simulink model "closedloop_saturation1"  (R2018a)
settings: Solver=ode23t  StartTime=0.0  StopTime=5  MaxStep=0.01  RelTol=1e-3
InitFcn:
  | % stop_time_as_str = get_param(gcs, 'StopTime');
  | % T= str2double(stop_time_as_str);
model workspace (MATLAB code in the model file):
  | % Simscape(TM) Multibody(TM) version: 7.1
  | 
  | % This is a model data file derived from a Simscape Multibody Import XML file using the smimport function.
  | % The data in this file sets the block parameter values in an imported Simscape Multibody model.
  | % For more information on this file, see the smimport function help page in the Simscape Multibody documentation.
  | % You can modify numerical values, but avoid any other changes to this file.
  | % Do not add code to this file. Do not edit the physical units shown in comments.
  | 
  | %%%VariableName:smiData
  | 
  | 
  | %============= RigidTransform =============%
  | 
  | %Initialize the RigidTransform structure array by filling in null values.
  | smiData.RigidTransform(23).translation = [0.0 0.0 0.0];
  | smiData.RigidTransform(23).angle = 0.0;
  | smiData.RigidTransform(23).axis = [0.0 0.0 0.0];
  | smiData.RigidTransform(23).ID = '';
  | 
  | %Translation Method - Cartesian
  | %Rotation Method - Arbitrary Axis
  | smiData.RigidTransform(1).translation = [0 0 20];  % mm
  | smiData.RigidTransform(1).angle = 3.1415926535897931;  % rad
  | smiData.RigidTransform(1).axis = [1 0 0];
  | smiData.RigidTransform(1).ID = 'B[Base-1:-:Plane-1]';
  | 
  | %Translation Method - Cartesian
  | %Rotation Method - Arbitrary Axis
  | smiData.RigidTransform(2).translation = [0 -280 30];  % mm
  | smiData.RigidTransform(2).angle = 3.1415926535897931;  % rad
  | smiData.RigidTransform(2).axis = [1 0 0];
  | smiData.RigidTransform(2).ID = 'F[Base-1:-:Plane-1]';
  | 
  | %Translation Method - Cartesian
  | %Rotation Method - Arbitrary Axis
  | smiData.RigidTransform(3).translation = [-650 -399.99999999999994 10];  % mm
  | smiData.RigidTransform(3).angle = 2.0943951023931953;  % rad
  | smiData.RigidTransform(3).axis = [0.57735026918962584 -0.57735026918962584 0.57735026918962584];
  | smiData.RigidTransform(3).ID = 'B[Plane-1:-:]';
  | 
  | %Translation Method - Cartesian
  | %Rotation Method - Arbitrary Axis
  | smiData.RigidTransform(4).translation = [-650 -119.99999999999994 0];  % mm
  | smiData.RigidTransform(4).angle = 2.0943951023931953;  % rad
  | smiData.RigidTransform(4).axis = [0.57735026918962584 -0.57735026918962584 0.57735026918962584];
  | smiData.RigidTransform(4).ID = 'F[Plane-1:-:]';
  | 
  | %Translation Method - Cartesian
  | %Rotation Method - Arbitrary Axis
  | smiData.RigidTransform(5).translation = [0 -20 60];  % mm
  | smiData.RigidTransform(5).angle = 2.0943951023931953;  % rad
  | smiData.RigidTransform(5).axis = [-0.57735026918962584 -0.57735026918962584 -0.57735026918962584];
  | smiData.RigidTransform(5).ID = 'B[Link1-1:-:Link2-1]';
  | 
  | %Translation Method - Cartesian
  | %Rotation Method - Arbitrary Axis
  | smiData.RigidTransform(6).translation = [20.000000000000004 -6.8922645368729718e-13 -40.000000000002252];  % mm
  | smiData.RigidTransform(6).angle = 2.0943951023931957;  % rad
  | smiData.RigidTransform(6).axis = [-0.57735026918962573 -0.57735026918962562 0.57735026918962573];
  | smiData.RigidTransform(6).ID = 'F[Link1-1:-:Link2-1]';
  | 
  | %Translation Method - Cartesian
  | %Rotation Method - Arbitrary Axis
  | smiData.RigidTransform(7).translation = [0 0 110.00000000000001];  % mm
  | smiData.RigidTransform(7).angle = 0;  % rad
  | smiData.RigidTransform(7).axis = [0 0 0];
  | smiData.RigidTransform(7).ID = 'B[Base-1:-:Link1-1]';
  | 
  | %Translation Method - Cartesian
  | %Rotation Method - Arbitrary Axis
  | smiData.RigidTransform(8).translation = [0 0 -2.8421709430404007e-14];  % mm
  | smiData.RigidTransform(8).angle = 0;  % rad
  | smiData.RigidTransform(8).axis = [0 0 0];
  | smiData.RigidTransform(8).ID = 'F[Base-1:-:Link1-1]';
  | 
  | %Translation Method - Cartesian
  | %Rotation Method - Arbitrary Axis
  | smiData.RigidTransform(9).translation = [-7 0 260];  % mm
  | smiData.RigidTransform(9).angle = 2.0943951023931953;  % rad
  | smiData.RigidTransform(9).axis = [0.57735026918962584 0.57735026918962584 0.57735026918962584];
  | smiData.RigidTransform(9).ID = 'B[Link2-1:-:Link3-1]';
  | 
  | %Translation Method - Cartesian
  | %Rotation Method - Arbitrary Axis
  | smiData.RigidTransform(10).translation = [7.0000000000000213 2.4034108037085389e-12 -40.000000000000242];  % mm
  | smiData.RigidTransform(10).angle = 2.0943951023931957;  % rad
  | smiData.RigidTransform(10).axis = [-0.57735026918962595 -0.57735026918962573 0.57735026918962551];
  | smiData.RigidTransform(10).ID = 'F[Link2-1:-:Link3-1]';
  | 
  | %Translation Method - Cartesian
  | %Rotation Method - Arbitrary Axis
  | smiData.RigidTransform(11).translation = [-12 0 220];  % mm
  | smiData.RigidTransform(11).angle = 2.0943951023931953;  % rad
  | smiData.RigidTransform(11).axis = [0.57735026918962584 0.57735026918962584 0.57735026918962584];
  | smiData.RigidTransform(11).ID = 'B[Link3-1:-:Link4-1]';
  | 
  | %Translation Method - Cartesian
  | %Rotation Method - Arbitrary Axis
  | smiData.RigidTransform(12).translation = [11.999999999999968 -3.5527136788005009e-14 -29.999999999999815];  % mm
  | smiData.RigidTransform(12).angle = 2.0943951023931957;  % rad
  | smiData.RigidTransform(12).axis = [-0.57735026918962573 -0.57735026918962573 0.57735026918962562];
  | smiData.RigidTransform(12).ID = 'F[Link3-1:-:Link4-1]';
  | 
  | %Translation Method - Cartesian
  | %Rotation Method - Arbitrary Axis
  | smiData.RigidTransform(13).translation = [0 0 0];  % mm
  | smiData.RigidTransform(13).angle = 0;  % rad
  | smiData.RigidTransform(13).axis = [0 0 0];
  | smiData.RigidTransform(13).ID = 'B[Base-1:-:]';
  | 
  | %Translation Method - Cartesian
  | %Rotation Method - Arbitrary Axis
  | smiData.RigidTransform(14).translation = [0 0 0];  % mm
  | smiData.RigidTransform(14).angle = 0;  % rad
  | smiData.RigidTransform(14).axis = [0 0 0];
  | smiData.RigidTransform(14).ID = 'F[Base-1:-:]';
  | 
  | %Translation Method - Cartesian
  | %Rotation Method - Arbitrary Axis
  | smiData.RigidTransform(15).translation = [0 1.1102230246251565e-13 20.000000000000018];  % mm
  | smiData.RigidTransform(15).angle = 0;  % rad
  | smiData.RigidTransform(15).axis = [0 0 0];
  | smiData.RigidTransform(15).ID = 'B[Link4-1:-:Tool1-1]';
  | 
  | %Translation Method - Cartesian
  | %Rotation Method - Arbitrary Axis
  | smiData.RigidTransform(16).translation = [2.4922286456785514e-12 -4.9999999999999751 1.2168044349891716e-13];  % mm
  | smiData.RigidTransform(16).angle = 2.0943951023931957;  % rad
  | smiData.RigidTransform(16).axis = [-0.57735026918962595 -0.57735026918962573 -0.57735026918962551];
  | smiData.RigidTransform(16).ID = 'F[Link4-1:-:Tool1-1]';
  | 
  | %Translation Method - Cartesian
  | %Rotation Method - Arbitrary Axis
  | smiData.RigidTransform(17).translation = [-40.385164807134494 17.000000000000028 2.5000000000000022];  % mm
  | smiData.RigidTransform(17).angle = 2.0943951023931953;  % rad
  | smiData.RigidTransform(17).axis = [0.57735026918962584 0.57735026918962584 0.57735026918962584];
  | smiData.RigidTransform(17).ID = 'B[Tool1-1:-:Tool2-1]';
  | 
  | %Translation Method - Cartesian
  | %Rotation Method - Arbitrary Axis
  | smiData.RigidTransform(18).translation = [-2.4999999999999627 10.385164807134508 -17.999999999999989];  % mm
  | smiData.RigidTransform(18).angle = 2.0943951023931957;  % rad
  | smiData.RigidTransform(18).axis = [0.57735026918962573 -0.57735026918962573 0.57735026918962562];
  | smiData.RigidTransform(18).ID = 'F[Tool1-1:-:Tool2-1]';
  | 
  | %Translation Method - Cartesian
  | %Rotation Method - Arbitrary Axis
  | smiData.RigidTransform(19).translation = [-40.385164807134494 15.000000000000014 -2.5000000000000022];  % mm
  | smiData.RigidTransform(19).angle = 2.0943951023931953;  % rad
  | smiData.RigidTransform(19).axis = [0.57735026918962584 0.57735026918962584 0.57735026918962584];
  | smiData.RigidTransform(19).ID = 'B[Tool1-1:-:Tool2-2]';
  | 
  | %Translation Method - Cartesian
  | %Rotation Method - Arbitrary Axis
  | smiData.RigidTransform(20).translation = [2.499999999999913 75.385164807134529 -19.99999999999995];  % mm
  | smiData.RigidTransform(20).angle = 2.0943951023931988;  % rad
  | smiData.RigidTransform(20).axis = [0.57735026918962384 -0.57735026918962662 0.57735026918962684];
  | smiData.RigidTransform(20).ID = 'F[Tool1-1:-:Tool2-2]';
  | 
  | %Translation Method - Cartesian
  | %Rotation Method - Arbitrary Axis
  | smiData.RigidTransform(21).translation = [0 0 0];  % mm
  | smiData.RigidTransform(21).angle = 0;  % rad
  | smiData.RigidTransform(21).axis = [0 0 0];
  | smiData.RigidTransform(21).ID = 'RootGround[Base-1]';
  | 
  | %Translation Method - Cartesian
  | %Rotation Method - Arbitrary Axis
  | smiData.RigidTransform(22).translation = [370 0 0];  % mm
  | smiData.RigidTransform(22).angle = 0;  % rad
  | smiData.RigidTransform(22).axis = [0 0 0];
  | smiData.RigidTransform(22).ID = 'SixDofRigidTransform[Box-1]';
  | 
  | %Translation Method - Cartesian
  | %Rotation Method - Arbitrary Axis
  | smiData.RigidTransform(23).translation = [370 130 20.000000000000004];  % mm
  | smiData.RigidTransform(23).angle = 1.5707963267948968;  % rad
  | smiData.RigidTransform(23).axis = [1 0 0];
  | smiData.RigidTransform(23).ID = 'SixDofRigidTransform[Box-2]';
  | 
  | 
  | %============= Solid =============%
  | %Center of Mass (CoM) %Moments of Inertia (MoI) %Product of Inertia (PoI)
  | 
  | %Initialize the Solid structure array by filling in null values.
  | smiData.Solid(9).mass = 0.0;
  | smiData.Solid(9).CoM = [0.0 0.0 0.0];
  | smiData.Solid(9).MoI = [0.0 0.0 0.0];
  | smiData.Solid(9).PoI = [0.0 0.0 0.0];
  | smiData.Solid(9).color = [0.0 0.0 0.0];
  | smiData.Solid(9).opacity = 0.0;
  | smiData.Solid(9).ID = '';
  | 
  | %Inertia Type - Custom
  | %Visual Properties - Simple
  | smiData.Solid(1).mass = 1.1003428269198252;  % kg
  | smiData.Solid(1).CoM = [0 0 49.154175588865094];  % mm
  | smiData.Solid(1).MoI = [2358.3181660426494 2358.318166042649 1952.1954924177403];  % kg*mm^2
  | smiData.Solid(1).PoI = [0 0 0];  % kg*mm^2
  | smiData.Solid(1).color = [1 0 0];
  | smiData.Solid(1).opacity = 1;
  | smiData.Solid(1).ID = 'Base*:*Default';
  | 
  | %Inertia Type - Custom
  | %Visual Properties - Simple
  | smiData.Solid(2).mass = 0.16090702237282686;  % kg
  | smiData.Solid(2).CoM = [0 0 24.735915171400126];  % mm
  | smiData.Solid(2).MoI = [100.06382794231057 98.635960389917443 84.94476439180923];  % kg*mm^2
  | smiData.Solid(2).PoI = [0 0 0];  % kg*mm^2
  | smiData.Solid(2).color = [1 1 0];
  | smiData.Solid(2).opacity = 1;
  | smiData.Solid(2).ID = 'Link1*:*Default';
  | 
  | %Inertia Type - Custom
  | %Visual Properties - Simple
  | smiData.Solid(3).mass = 0.2437115568304318;  % kg
  | smiData.Solid(3).CoM = [0 0 110];  % mm
  | smiData.Solid(3).MoI = [1435.7626334656898 1433.8027139688336 35.317093070443498];  % kg*mm^2
  | smiData.Solid(3).PoI = [0 0 0];  % kg*mm^2
  | smiData.Solid(3).color = [0 1 0];
  | smiData.Solid(3).opacity = 1;
  | smiData.Solid(3).ID = 'Link2*:*Default';
  | 
  | %Inertia Type - Custom
  | %Visual Properties - Simple
  | smiData.Solid(4).mass = 0.20371288755859771;  % kg
  | smiData.Solid(4).CoM = [0 0 90.000000000000028];  % mm
  | smiData.Solid(4).MoI = [838.71368172462144 838.57689215918276 30.87485985708695];  % kg*mm^2
  | smiData.Solid(4).PoI = [0 0 0];  % kg*mm^2
  | smiData.Solid(4).color = [0.75294117647058822 0 0];
  | smiData.Solid(4).opacity = 1;
  | smiData.Solid(4).ID = 'Link3*:*Default';
  | 
  | %Inertia Type - Custom
  | %Visual Properties - Simple
  | smiData.Solid(5).mass = 0.034520000161264247;  % kg
  | smiData.Solid(5).CoM = [0 0 1.6273478174011298];  % mm
  | smiData.Solid(5).MoI = [12.290203304115773 11.522708446040582 4.7230757356872166];  % kg*mm^2
  | smiData.Solid(5).PoI = [0 0 0];  % kg*mm^2
  | smiData.Solid(5).color = [0 0 1];
  | smiData.Solid(5).opacity = 1;
  | smiData.Solid(5).ID = 'Link4*:*Default';
  | 
  | %Inertia Type - Custom
  | %Visual Properties - Simple
  | smiData.Solid(6).mass = 0.027022897183705957;  % kg
  | smiData.Solid(6).CoM = [0 8.7345746780211826 0];  % mm
  | smiData.Solid(6).MoI = [3.5333125191281254 9.7891180754786511 7.6676875191281253];  % kg*mm^2
  | smiData.Solid(6).PoI = [0 0 0];  % kg*mm^2
  | smiData.Solid(6).color = [0.25098039215686274 0.25098039215686274 0.25098039215686274];
  | smiData.Solid(6).opacity = 1;
  | smiData.Solid(6).ID = 'Tool1*:*Default';
  | 
  | %Inertia Type - Custom
  | %Visual Properties - Simple
  | smiData.Solid(7).mass = 0.0079500000000000022;  % kg
  | smiData.Solid(7).CoM = [0 2.5 0.11949685534591241];  % mm
  | smiData.Solid(7).MoI = [1.0650489779874213 2.1150489779874211 1.0831250000000001];  % kg*mm^2
  | smiData.Solid(7).PoI = [0 0 0];  % kg*mm^2
  | smiData.Solid(7).color = [1 1 1];
  | smiData.Solid(7).opacity = 1;
  | smiData.Solid(7).ID = 'Tool2*:*Default';
  | 
  | %Inertia Type - Custom
  | %Visual Properties - Simple
  | smiData.Solid(8).mass = 18.351953541323557;  % kg
  | smiData.Solid(8).CoM = [0 87.205525821856682 28.801664490507051];  % mm
  | smiData.Solid(8).MoI = [779908.52114150906 1591376.3808165451 2330810.8044516048];  % kg*mm^2
  | smiData.Solid(8).PoI = [-49463.262725423032 0 0];  % kg*mm^2
  | smiData.Solid(8).color = [0.75294117647058822 1 1];
  | smiData.Solid(8).opacity = 1;
  | smiData.Solid(8).ID = 'Plane*:*Default';
  | 
  | %Inertia Type - Custom
  | %Visual Properties - Simple
  | smiData.Solid(9).mass = 0.064000000000000015;  % kg
  | smiData.Solid(9).CoM = [0 0 20];  % mm
  | smiData.Solid(9).MoI = [17.066666666666666 17.066666666666666 17.066666666666666];  % kg*mm^2
  | smiData.Solid(9).PoI = [0 0 0];  % kg*mm^2
  | smiData.Solid(9).color = [0.90980392156862744 0.44313725490196076 0.031372549019607843];
  | smiData.Solid(9).opacity = 1;
  | smiData.Solid(9).ID = 'Box*:*Default';
  | 
  | 
  | %============= Joint =============%
  | %X Revolute Primitive (Rx) %Y Revolute Primitive (Ry) %Z Revolute Primitive (Rz)
  | %X Prismatic Primitive (Px) %Y Prismatic Primitive (Py) %Z Prismatic Primitive (Pz) %Spherical Primitive (S)
  | %Constant Velocity Primitive (CV) %Lead Screw Primitive (LS)
  | %Position Target (Pos)
  | 
  | %Initialize the PrismaticJoint structure array by filling in null values.
  | smiData.PrismaticJoint(2).Pz.Pos = 0.0;
  | smiData.PrismaticJoint(2).ID = '';
  | 
  | smiData.PrismaticJoint(1).Pz.Pos = 0;  % m
  | smiData.PrismaticJoint(1).ID = '[Tool1-1:-:Tool2-1]';
  | 
  | smiData.PrismaticJoint(2).Pz.Pos = 0;  % m
  | smiData.PrismaticJoint(2).ID = '[Tool1-1:-:Tool2-2]';
  | 
  | 
  | %Initialize the RevoluteJoint structure array by filling in null values.
  | smiData.RevoluteJoint(6).Rz.Pos = 0.0;
  | smiData.RevoluteJoint(6).ID = '';
  | 
  | smiData.RevoluteJoint(1).Rz.Pos = 0;  % deg
  | smiData.RevoluteJoint(1).ID = '[Base-1:-:Plane-1]';
  | 
  | smiData.RevoluteJoint(2).Rz.Pos = 122.57056361367474;  % deg
  | smiData.RevoluteJoint(2).ID = '[Link1-1:-:Link2-1]';
  | 
  | smiData.RevoluteJoint(3).Rz.Pos = 0;  % deg
  | smiData.RevoluteJoint(3).ID = '[Base-1:-:Link1-1]';
  | 
  | smiData.RevoluteJoint(4).Rz.Pos = 69.246638981667132;  % deg
  | smiData.RevoluteJoint(4).ID = '[Link2-1:-:Link3-1]';
  | 
  | smiData.RevoluteJoint(5).Rz.Pos = 179.99999999999991;  % deg
  | smiData.RevoluteJoint(5).ID = '[Link3-1:-:Link4-1]';
  | 
  | smiData.RevoluteJoint(6).Rz.Pos = 90.000000000000028;  % deg
  | smiData.RevoluteJoint(6).ID = '[Link4-1:-:Tool1-1]';
values from neighbouring files (symbols this model uses):
  m = t/T    [JointTraj_1deg.m]    (also in JointTraj_3deg.m = 3*(t/T)^2-2*(t/T)^3; Line_CartesianTr.m = 3*(t/T)^2-2*(t/T)^3; circleTraj.m = 3*(t/T)^2-2*(t/T)^3; circleTraj45.m = 3*(t/T)^2-2*(t/T)^3)
undefined symbols (not defined in the file or in its folder): smiData, X, Y, Z
libraries: sm_lib x55, nesl_utility x18, simulink x4
(part 1 of 2)
settings Model: Creator=AA_M991  LastModifiedBy=Yara
settings DataIOCC: ReturnWorkspaceOutputs=on
settings SFSimCC: SimUseLocalCustomCode=on
settings RTWCC: RTWUseLocalCustomCode=on

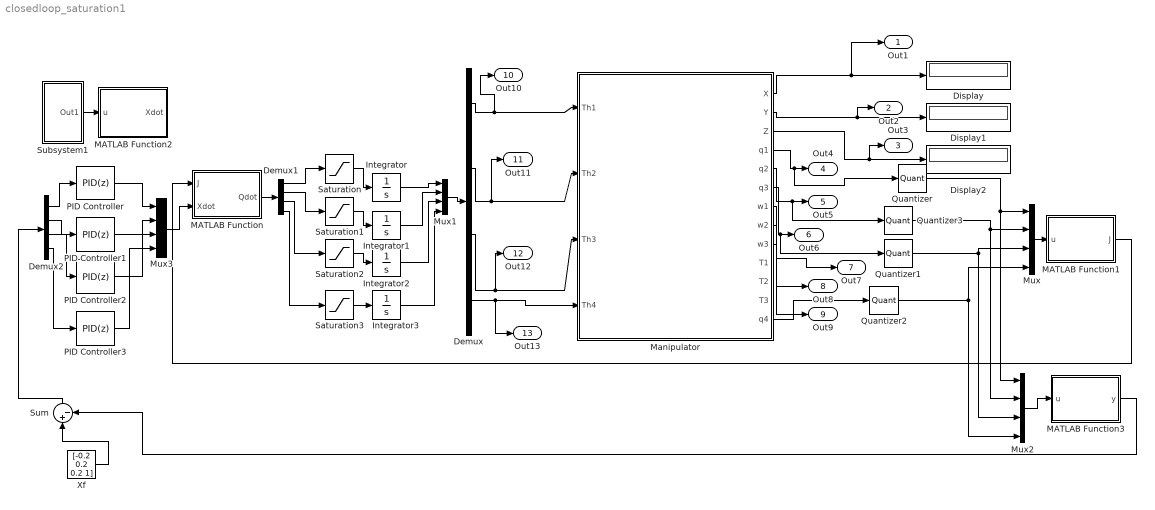
== system closedloop_saturation1 ==
  Demux : Demux
  Demux1 : Demux
  Demux2 : Demux
  Display : Display
  Display1 : Display
  Display2 : Display
  Integrator : Integrator
  Integrator1 : Integrator  InitialCondition=pi/3
  Integrator2 : Integrator  InitialCondition=-pi/3
  Integrator3 : Integrator
  MATLAB Function : MATLAB Function  TreatAsAtomicUnit=on
  MATLAB Function1 : MATLAB Function  TreatAsAtomicUnit=on
  MATLAB Function2 : MATLAB Function  TreatAsAtomicUnit=on
  MATLAB Function3 : MATLAB Function  TreatAsAtomicUnit=on
  Manipulator : Subsystem  mask{Th0=0, Th1=pi/4, Th2=-pi/4}
      mask prompts: Th2 "Th3"
      mask Display: %image('icon.PNG'); % Use "Edit Image" on toolstrip to change.
  Mux{,1..3} (4 alike) : Mux
  PID Controller : simulink/Continuous/PID Controller  Controller=PID  TimeDomain=Discrete-time  SampleTime=-1  IntegratorMethod=Forward Euler  FilterMethod=Forward Euler  Form=Parallel  UseFilter=on  ControllerParametersSource=internal  P=1  I=0  D=0.1  N=6.065  InitialConditionSource=internal  InitialConditionForIntegrator=0  InitialConditionForFilter=0  ExternalReset=none  LimitOutput=off  UpperSaturationLimit=inf  LowerSaturationLimit=-inf  LinearizeAsGain=on  AntiWindupMode=none  Kb=1  TrackingMode=off  Kt=1  PParamMin=[]  PParamMax=[]  IParamMin=[]  IParamMax=[]  DParamMin=[]  DParamMax=[]  NParamMin=[]  NParamMax=[]  KbParamMin=[]  KbParamMax=[]  KtParamMin=[]  KtParamMax=[]  POutMin=[]  POutMax=[]  IOutMin=[]  IOutMax=[]  DOutMin=[]  DOutMax=[]  NOutMin=[]  NOutMax=[]  KbOutMin=[]  KbOutMax=[]  KtOutMin=[]  KtOutMax=[]  IntegratorOutMin=[]  IntegratorOutMax=[]  FilterOutMin=[]  FilterOutMax=[]  SumOutMin=[]  SumOutMax=[]  SumI1OutMin=[]  SumI1OutMax=[]  SumI2OutMin=[]  SumI2OutMax=[]  SumI3OutMin=[]  SumI3OutMax=[]  SumDOutMin=[]  SumDOutMax=[]  SaturationOutMin=[]  SaturationOutMax=[]  IntegratorContinuousStateAttributes=''  IntegratorStateMustResolveToSignalObject=off  IntegratorRTWStateStorageClass=Auto  FilterContinuousStateAttributes=''  FilterStateMustResolveToSignalObject=off  FilterRTWStateStorageClass=Auto  DifferentiatorICPrevScaledInput=0  DifferentiatorOutMin=[]  DifferentiatorOutMax=[]  FilterDiffOutCoefMin=[]  FilterDiffOutCoefMax=[]  SumDenOutMin=[]  SumDenOutMax=[]  SumNumOutMin=[]  SumNumOutMax=[]  ReciprocalOutMin=[]  ReciprocalOutMax=[]  DivideOutMin=[]  DivideOutMax=[]  TunerSelectOption=Transfer Function Based (PID Tuner App)
  PID Controller1 : simulink/Continuous/PID Controller  Controller=PID  TimeDomain=Discrete-time  SampleTime=-1  IntegratorMethod=Forward Euler  FilterMethod=Forward Euler  Form=Parallel  UseFilter=on  ControllerParametersSource=internal  P=1  I=0  D=0.1  N=119.3  InitialConditionSource=internal  InitialConditionForIntegrator=0  InitialConditionForFilter=0  ExternalReset=none  LimitOutput=off  UpperSaturationLimit=inf  LowerSaturationLimit=-inf  LinearizeAsGain=on  AntiWindupMode=none  Kb=1  TrackingMode=off  Kt=1  PParamMin=[]  PParamMax=[]  IParamMin=[]  IParamMax=[]  DParamMin=[]  DParamMax=[]  NParamMin=[]  NParamMax=[]  KbParamMin=[]  KbParamMax=[]  KtParamMin=[]  KtParamMax=[]  POutMin=[]  POutMax=[]  IOutMin=[]  IOutMax=[]  DOutMin=[]  DOutMax=[]  NOutMin=[]  NOutMax=[]  KbOutMin=[]  KbOutMax=[]  KtOutMin=[]  KtOutMax=[]  IntegratorOutMin=[]  IntegratorOutMax=[]  FilterOutMin=[]  FilterOutMax=[]  SumOutMin=[]  SumOutMax=[]  SumI1OutMin=[]  SumI1OutMax=[]  SumI2OutMin=[]  SumI2OutMax=[]  SumI3OutMin=[]  SumI3OutMax=[]  SumDOutMin=[]  SumDOutMax=[]  SaturationOutMin=[]  SaturationOutMax=[]  IntegratorContinuousStateAttributes=''  IntegratorStateMustResolveToSignalObject=off  IntegratorRTWStateStorageClass=Auto  FilterContinuousStateAttributes=''  FilterStateMustResolveToSignalObject=off  FilterRTWStateStorageClass=Auto  DifferentiatorICPrevScaledInput=0  DifferentiatorOutMin=[]  DifferentiatorOutMax=[]  FilterDiffOutCoefMin=[]  FilterDiffOutCoefMax=[]  SumDenOutMin=[]  SumDenOutMax=[]  SumNumOutMin=[]  SumNumOutMax=[]  ReciprocalOutMin=[]  ReciprocalOutMax=[]  DivideOutMin=[]  DivideOutMax=[]  TunerSelectOption=Transfer Function Based (PID Tuner App)
  PID Controller2 : simulink/Continuous/PID Controller  Controller=PID  TimeDomain=Discrete-time  SampleTime=-1  IntegratorMethod=Forward Euler  FilterMethod=Forward Euler  Form=Parallel  UseFilter=on  ControllerParametersSource=internal  P=1  I=0  D=0.1  N=12.87  InitialConditionSource=internal  InitialConditionForIntegrator=0  InitialConditionForFilter=0  ExternalReset=none  LimitOutput=off  UpperSaturationLimit=inf  LowerSaturationLimit=-inf  LinearizeAsGain=on  AntiWindupMode=none  Kb=1  TrackingMode=off  Kt=1  PParamMin=[]  PParamMax=[]  IParamMin=[]  IParamMax=[]  DParamMin=[]  DParamMax=[]  NParamMin=[]  NParamMax=[]  KbParamMin=[]  KbParamMax=[]  KtParamMin=[]  KtParamMax=[]  POutMin=[]  POutMax=[]  IOutMin=[]  IOutMax=[]  DOutMin=[]  DOutMax=[]  NOutMin=[]  NOutMax=[]  KbOutMin=[]  KbOutMax=[]  KtOutMin=[]  KtOutMax=[]  IntegratorOutMin=[]  IntegratorOutMax=[]  FilterOutMin=[]  FilterOutMax=[]  SumOutMin=[]  SumOutMax=[]  SumI1OutMin=[]  SumI1OutMax=[]  SumI2OutMin=[]  SumI2OutMax=[]  SumI3OutMin=[]  SumI3OutMax=[]  SumDOutMin=[]  SumDOutMax=[]  SaturationOutMin=[]  SaturationOutMax=[]  IntegratorContinuousStateAttributes=''  IntegratorStateMustResolveToSignalObject=off  IntegratorRTWStateStorageClass=Auto  FilterContinuousStateAttributes=''  FilterStateMustResolveToSignalObject=off  FilterRTWStateStorageClass=Auto  DifferentiatorICPrevScaledInput=0  DifferentiatorOutMin=[]  DifferentiatorOutMax=[]  FilterDiffOutCoefMin=[]  FilterDiffOutCoefMax=[]  SumDenOutMin=[]  SumDenOutMax=[]  SumNumOutMin=[]  SumNumOutMax=[]  ReciprocalOutMin=[]  ReciprocalOutMax=[]  DivideOutMin=[]  DivideOutMax=[]  TunerSelectOption=Transfer Function Based (PID Tuner App)
  PID Controller3 : simulink/Continuous/PID Controller  Controller=PID  TimeDomain=Discrete-time  SampleTime=-1  IntegratorMethod=Forward Euler  FilterMethod=Forward Euler  Form=Parallel  UseFilter=on  ControllerParametersSource=internal  P=1  I=0  D=0.1  N=1.706  InitialConditionSource=internal  InitialConditionForIntegrator=0  InitialConditionForFilter=0  ExternalReset=none  LimitOutput=off  UpperSaturationLimit=inf  LowerSaturationLimit=-inf  LinearizeAsGain=on  AntiWindupMode=none  Kb=1  TrackingMode=off  Kt=1  PParamMin=[]  PParamMax=[]  IParamMin=[]  IParamMax=[]  DParamMin=[]  DParamMax=[]  NParamMin=[]  NParamMax=[]  KbParamMin=[]  KbParamMax=[]  KtParamMin=[]  KtParamMax=[]  POutMin=[]  POutMax=[]  IOutMin=[]  IOutMax=[]  DOutMin=[]  DOutMax=[]  NOutMin=[]  NOutMax=[]  KbOutMin=[]  KbOutMax=[]  KtOutMin=[]  KtOutMax=[]  IntegratorOutMin=[]  IntegratorOutMax=[]  FilterOutMin=[]  FilterOutMax=[]  SumOutMin=[]  SumOutMax=[]  SumI1OutMin=[]  SumI1OutMax=[]  SumI2OutMin=[]  SumI2OutMax=[]  SumI3OutMin=[]  SumI3OutMax=[]  SumDOutMin=[]  SumDOutMax=[]  SaturationOutMin=[]  SaturationOutMax=[]  IntegratorContinuousStateAttributes=''  IntegratorStateMustResolveToSignalObject=off  IntegratorRTWStateStorageClass=Auto  FilterContinuousStateAttributes=''  FilterStateMustResolveToSignalObject=off  FilterRTWStateStorageClass=Auto  DifferentiatorICPrevScaledInput=0  DifferentiatorOutMin=[]  DifferentiatorOutMax=[]  FilterDiffOutCoefMin=[]  FilterDiffOutCoefMax=[]  SumDenOutMin=[]  SumDenOutMax=[]  SumNumOutMin=[]  SumNumOutMax=[]  ReciprocalOutMin=[]  ReciprocalOutMax=[]  DivideOutMin=[]  DivideOutMax=[]  TunerSelectOption=Transfer Function Based (PID Tuner App)
  Quantizer{,1..3} (4 alike) : Quantizer  QuantizationInterval=0.0087
  Saturation{,1..3} (4 alike) : Saturate  UpperLimit=1  LowerLimit=-1
  Subsystem1 : Subsystem
  Sum : Sum  Inputs=|+-
  Xf : Constant  Value=[-0.2 0.2 0.2 1]
  Out1 : Outport
  Out2 : Outport  Port=2
  Out3 : Outport  Port=3
  Out4 : Outport  Port=4
  Out5 : Outport  Port=5
  Out6 : Outport  Port=6
  Out7 : Outport  Port=7
  Out8 : Outport  Port=8
  Out9 : Outport  Port=9
  Out10 : Outport  Port=10
  Out11 : Outport  Port=11
  Out12 : Outport  Port=12
  Out13 : Outport  Port=13
  wires:
  MATLAB Function/1(Qdot) -> Demux1/1
  Demux/3 -> Out12/1, Manipulator/3(Th3)
  Mux/1 -> MATLAB Function1/1(u)
  Saturation2/1 -> Integrator2/1
  Subsystem1/1(Out1) -> MATLAB Function2/1(u)
  Manipulator/5(q2) -> Quantizer3/1, Out5/1
  Demux2/4 -> PID Controller3/1
  PID Controller/1 -> Mux3/1
  PID Controller3/1 -> Mux3/4
  Quantizer2/1 -> Mux2/4, Mux/4
  Saturation1/1 -> Integrator1/1
  Demux1/1 -> Saturation/1
  Manipulator/6(q3) -> Quantizer1/1, Out6/1
  Demux/1 -> Out10/1, Manipulator/1(Th1)
  Integrator/1 -> Mux1/1
  Quantizer3/1 -> Mux2/2, Mux/2
  Manipulator/4(q1) -> Quantizer/1, Out4/1
  MATLAB Function3/1(y) -> Sum/2
  MATLAB Function1/1(J) -> MATLAB Function/1(J)
  PID Controller2/1 -> Mux3/3
  Mux3/1 -> MATLAB Function/2(Xdot)
  Saturation3/1 -> Integrator3/1
  Demux2/1 -> PID Controller/1
  Saturation/1 -> Integrator/1
  Manipulator/8(w2) -> Out8/1
  Mux1/1 -> Demux/1
  Mux2/1 -> MATLAB Function3/1(u)
  Manipulator/13(q4) -> Quantizer2/1
  Quantizer/1 -> Mux/1, Mux2/1
  Demux2/2 -> PID Controller1/1
  PID Controller1/1 -> Mux3/2
  Sum/1 -> Demux2/1
  Demux/4 -> Out13/1, Manipulator/4(Th4)
  Manipulator/3(Z) -> Out3/1, Display2/1
  Quantizer1/1 -> Mux/3, Mux2/3
  Demux/2 -> Out11/1, Manipulator/2(Th2)
  Demux1/3 -> Saturation2/1
  Manipulator/1(X) -> Out1/1, Display/1
  Manipulator/9(w3) -> Out9/1
  Manipulator/2(Y) -> Out2/1, Display1/1
  Manipulator/7(w1) -> Out7/1
  Demux1/2 -> Saturation1/1
  Xf/1 -> Sum/1
  Integrator1/1 -> Mux1/2
  Integrator2/1 -> Mux1/3
  Demux1/4 -> Saturation3/1
  Demux2/3 -> PID Controller2/1
  Integrator3/1 -> Mux1/4

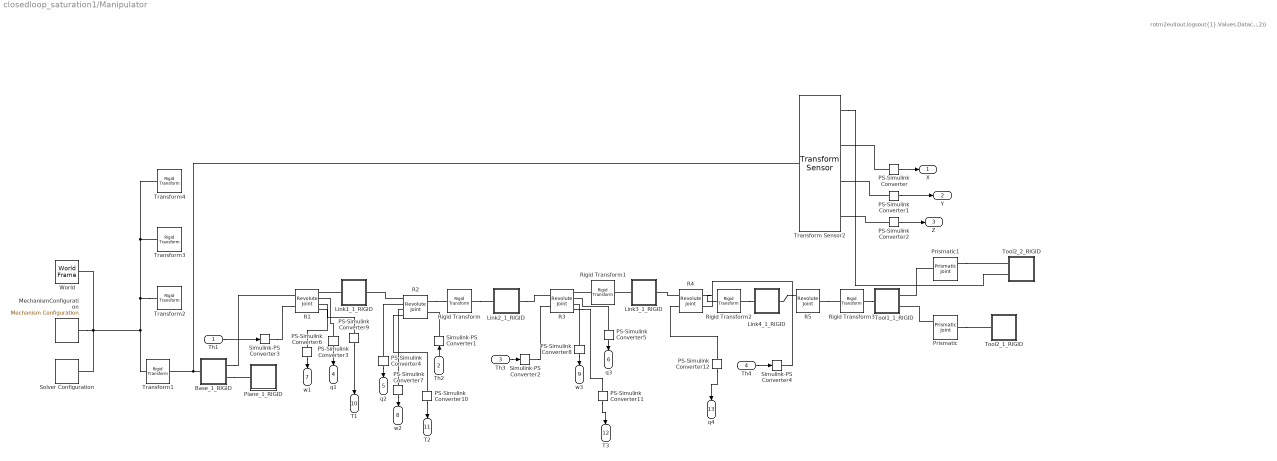
== system closedloop_saturation1/Manipulator ==
  note: rotm2eul(out.logsout{1}.Values.Data(:,:,2))
  Th1 : Inport
  Th2 : Inport  Port=2
  Th3 : Inport  Port=3
  Th4 : Inport  Port=4
  Base_1_RIGID : Subsystem
  Link1_1_RIGID : Subsystem
  Link2_1_RIGID : Subsystem
  Link3_1_RIGID : Subsystem
  Link4_1_RIGID : Subsystem
  MechanismConfiguration : sm_lib/Utilities/Mechanism Configuration  UniformGravity=Constant  GravityVector=[0 0 -9.81]  GravityUnits=m/s^2  LinearizationDelta=0.001
  PS-Simulink Converter : nesl_utility/PS-Simulink Converter  PhysicalDomain=network_engine_domain  SubClassName=ps_output  LeftPortType=input  RightPortType=output  PseudoPeriodic=off  Frequencies=[]  Unit=m  AffineConversion=off
  PS-Simulink Converter1 : nesl_utility/PS-Simulink Converter  PhysicalDomain=network_engine_domain  SubClassName=ps_output  LeftPortType=input  RightPortType=output  PseudoPeriodic=off  Frequencies=[]  Unit=m  AffineConversion=off
  PS-Simulink Converter10 : nesl_utility/PS-Simulink Converter  PhysicalDomain=network_engine_domain  SubClassName=ps_output  LeftPortType=input  RightPortType=output  PseudoPeriodic=off  Frequencies=[]  Unit=N*m  AffineConversion=off
  PS-Simulink Converter11 : nesl_utility/PS-Simulink Converter  PhysicalDomain=network_engine_domain  SubClassName=ps_output  LeftPortType=input  RightPortType=output  PseudoPeriodic=off  Frequencies=[]  Unit=N*m  AffineConversion=off
  PS-Simulink Converter{3..5,12} (4 alike) : nesl_utility/PS-Simulink Converter  PhysicalDomain=network_engine_domain  SubClassName=ps_output  LeftPortType=input  RightPortType=output  PseudoPeriodic=off  Frequencies=[]  Unit=rad  AffineConversion=off
  PS-Simulink Converter2 : nesl_utility/PS-Simulink Converter  PhysicalDomain=network_engine_domain  SubClassName=ps_output  LeftPortType=input  RightPortType=output  PseudoPeriodic=off  Frequencies=[]  Unit=m  AffineConversion=off
  PS-Simulink Converter6 : nesl_utility/PS-Simulink Converter  PhysicalDomain=network_engine_domain  SubClassName=ps_output  LeftPortType=input  RightPortType=output  PseudoPeriodic=off  Frequencies=[]  Unit=rad/s  AffineConversion=off
  PS-Simulink Converter7 : nesl_utility/PS-Simulink Converter  PhysicalDomain=network_engine_domain  SubClassName=ps_output  LeftPortType=input  RightPortType=output  PseudoPeriodic=off  Frequencies=[]  Unit=rad/s  AffineConversion=off
  PS-Simulink Converter8 : nesl_utility/PS-Simulink Converter  PhysicalDomain=network_engine_domain  SubClassName=ps_output  LeftPortType=input  RightPortType=output  PseudoPeriodic=off  Frequencies=[]  Unit=rad/s  AffineConversion=off
  PS-Simulink Converter9 : nesl_utility/PS-Simulink Converter  PhysicalDomain=network_engine_domain  SubClassName=ps_output  LeftPortType=input  RightPortType=output  PseudoPeriodic=off  Frequencies=[]  Unit=N*m  AffineConversion=off
  Plane_1_RIGID : Subsystem
  Prismatic : sm_lib/Joints/Prismatic Joint  SenseConstraintForce=off  SenseConstraintForceX=off  SenseConstraintForceY=off  SenseConstraintForceZ=off  SenseConstraintTorque=off  SenseConstraintTorqueX=off  SenseConstraintTorqueY=off  SenseConstraintTorqueZ=off  SenseTotalForce=off  SenseTotalForceX=off  SenseTotalForceY=off  SenseTotalForceZ=off  SenseTotalTorque=off  SenseTotalTorqueX=off  SenseTotalTorqueY=off  SenseTotalTorqueZ=off  CompositeWrenchDir=FollowerOnBase  CompositeWrenchFrame=BaseFrame  EquilibriumPosition=0  EquilibriumPositionUnits=m  SpringStiffness=0  SpringStiffnessUnits=N/m  DampingCoefficient=0  DampingCoefficientUnits=N/(m/s)  TorqueActuationMode=ComputedTorque  MotionActuationMode=InputMotion  SensePosition=off  SenseVelocity=off  SenseAcceleration=off  SenseTorqueForce=off  PositionTargetSpecify=on  PositionTargetPriority=Low  PositionTargetValue=0  PositionTargetValueUnits=m  VelocityTargetSpecify=off  VelocityTargetPriority=High  VelocityTargetValue=0.1  VelocityTargetValueUnits=m/s
  Prismatic1 : sm_lib/Joints/Prismatic Joint  SenseConstraintForce=off  SenseConstraintForceX=off  SenseConstraintForceY=off  SenseConstraintForceZ=off  SenseConstraintTorque=off  SenseConstraintTorqueX=off  SenseConstraintTorqueY=off  SenseConstraintTorqueZ=off  SenseTotalForce=off  SenseTotalForceX=off  SenseTotalForceY=off  SenseTotalForceZ=off  SenseTotalTorque=off  SenseTotalTorqueX=off  SenseTotalTorqueY=off  SenseTotalTorqueZ=off  CompositeWrenchDir=FollowerOnBase  CompositeWrenchFrame=BaseFrame  EquilibriumPosition=0  EquilibriumPositionUnits=m  SpringStiffness=0  SpringStiffnessUnits=N/m  DampingCoefficient=0  DampingCoefficientUnits=N/(m/s)  TorqueActuationMode=ComputedTorque  MotionActuationMode=InputMotion  SensePosition=off  SenseVelocity=off  SenseAcceleration=off  SenseTorqueForce=off  PositionTargetSpecify=on  PositionTargetPriority=Low  PositionTargetValue=0  PositionTargetValueUnits=m  VelocityTargetSpecify=off  VelocityTargetPriority=High  VelocityTargetValue=0.1  VelocityTargetValueUnits=m/s
  R1 : sm_lib/Joints/Revolute Joint  SenseConstraintForce=off  SenseConstraintForceX=off  SenseConstraintForceY=off  SenseConstraintForceZ=off  SenseConstraintTorque=off  SenseConstraintTorqueX=off  SenseConstraintTorqueY=off  SenseConstraintTorqueZ=off  SenseTotalForce=off  SenseTotalForceX=off  SenseTotalForceY=off  SenseTotalForceZ=off  SenseTotalTorque=off  SenseTotalTorqueX=off  SenseTotalTorqueY=off  SenseTotalTorqueZ=off  CompositeWrenchDir=FollowerOnBase  CompositeWrenchFrame=BaseFrame  EquilibriumPosition=0  EquilibriumPositionUnits=rad  SpringStiffness=0  SpringStiffnessUnits=N*m/rad  DampingCoefficient=0  DampingCoefficientUnits=N*m/(rad/s)  TorqueActuationMode=ComputedTorque  MotionActuationMode=InputMotion  SensePosition=on  SenseVelocity=on  SenseAcceleration=off  SenseTorqueForce=on  PositionTargetSpecify=on  PositionTargetPriority=Low  PositionTargetValue=Th0  PositionTargetValueUnits=rad  VelocityTargetSpecify=off  VelocityTargetPriority=High  VelocityTargetValue=0  VelocityTargetValueUnits=deg/s
  R2 : sm_lib/Joints/Revolute Joint  SenseConstraintForce=off  SenseConstraintForceX=off  SenseConstraintForceY=off  SenseConstraintForceZ=off  SenseConstraintTorque=off  SenseConstraintTorqueX=off  SenseConstraintTorqueY=off  SenseConstraintTorqueZ=off  SenseTotalForce=off  SenseTotalForceX=off  SenseTotalForceY=off  SenseTotalForceZ=off  SenseTotalTorque=off  SenseTotalTorqueX=off  SenseTotalTorqueY=off  SenseTotalTorqueZ=off  CompositeWrenchDir=FollowerOnBase  CompositeWrenchFrame=BaseFrame  EquilibriumPosition=0  EquilibriumPositionUnits=rad  SpringStiffness=0  SpringStiffnessUnits=N*m/rad  DampingCoefficient=0  DampingCoefficientUnits=N*m/(rad/s)  TorqueActuationMode=ComputedTorque  MotionActuationMode=InputMotion  SensePosition=on  SenseVelocity=on  SenseAcceleration=off  SenseTorqueForce=on  PositionTargetSpecify=on  PositionTargetPriority=Low  PositionTargetValue=Th1  PositionTargetValueUnits=rad  VelocityTargetSpecify=off  VelocityTargetPriority=High  VelocityTargetValue=0  VelocityTargetValueUnits=deg/s
  R3 : sm_lib/Joints/Revolute Joint  SenseConstraintForce=off  SenseConstraintForceX=off  SenseConstraintForceY=off  SenseConstraintForceZ=off  SenseConstraintTorque=off  SenseConstraintTorqueX=off  SenseConstraintTorqueY=off  SenseConstraintTorqueZ=off  SenseTotalForce=off  SenseTotalForceX=off  SenseTotalForceY=off  SenseTotalForceZ=off  SenseTotalTorque=off  SenseTotalTorqueX=off  SenseTotalTorqueY=off  SenseTotalTorqueZ=off  CompositeWrenchDir=FollowerOnBase  CompositeWrenchFrame=BaseFrame  EquilibriumPosition=0  EquilibriumPositionUnits=deg  SpringStiffness=0  SpringStiffnessUnits=N*m/rad  DampingCoefficient=0  DampingCoefficientUnits=N*m/(rad/s)  TorqueActuationMode=ComputedTorque  MotionActuationMode=InputMotion  SensePosition=on  SenseVelocity=on  SenseAcceleration=off  SenseTorqueForce=on  PositionTargetSpecify=on  PositionTargetPriority=High  PositionTargetValue=Th2  PositionTargetValueUnits=rad  VelocityTargetSpecify=off  VelocityTargetPriority=High  VelocityTargetValue=0  VelocityTargetValueUnits=deg/s
  R4 : sm_lib/Joints/Revolute Joint  SenseConstraintForce=off  SenseConstraintForceX=off  SenseConstraintForceY=off  SenseConstraintForceZ=off  SenseConstraintTorque=off  SenseConstraintTorqueX=off  SenseConstraintTorqueY=off  SenseConstraintTorqueZ=off  SenseTotalForce=off  SenseTotalForceX=off  SenseTotalForceY=off  SenseTotalForceZ=off  SenseTotalTorque=off  SenseTotalTorqueX=off  SenseTotalTorqueY=off  SenseTotalTorqueZ=off  CompositeWrenchDir=FollowerOnBase  CompositeWrenchFrame=BaseFrame  EquilibriumPosition=0  EquilibriumPositionUnits=rad  SpringStiffness=0  SpringStiffnessUnits=N*m/rad  DampingCoefficient=0  DampingCoefficientUnits=N*m/(rad/s)  TorqueActuationMode=ComputedTorque  MotionActuationMode=InputMotion  SensePosition=on  SenseVelocity=off  SenseAcceleration=off  SenseTorqueForce=off  PositionTargetSpecify=on  PositionTargetPriority=Low  PositionTargetValue=0  PositionTargetValueUnits=deg  VelocityTargetSpecify=off  VelocityTargetPriority=High  VelocityTargetValue=0  VelocityTargetValueUnits=deg/s
  R5 : sm_lib/Joints/Revolute Joint  SenseConstraintForce=off  SenseConstraintForceX=off  SenseConstraintForceY=off  SenseConstraintForceZ=off  SenseConstraintTorque=off  SenseConstraintTorqueX=off  SenseConstraintTorqueY=off  SenseConstraintTorqueZ=off  SenseTotalForce=off  SenseTotalForceX=off  SenseTotalForceY=off  SenseTotalForceZ=off  SenseTotalTorque=off  SenseTotalTorqueX=off  SenseTotalTorqueY=off  SenseTotalTorqueZ=off  CompositeWrenchDir=FollowerOnBase  CompositeWrenchFrame=BaseFrame  EquilibriumPosition=0  EquilibriumPositionUnits=rad  SpringStiffness=0  SpringStiffnessUnits=N*m/rad  DampingCoefficient=0  DampingCoefficientUnits=N*m/(rad/s)  TorqueActuationMode=ComputedTorque  MotionActuationMode=InputMotion  SensePosition=off  SenseVelocity=off  SenseAcceleration=off  SenseTorqueForce=off  PositionTargetSpecify=on  PositionTargetPriority=Low  PositionTargetValue=0  PositionTargetValueUnits=deg  VelocityTargetSpecify=off  VelocityTargetPriority=High  VelocityTargetValue=0  VelocityTargetValueUnits=deg/s
  Rigid Transform : sm_lib/Frames and Transforms/Rigid Transform  TranslationMethod=None  TranslationStandardOffset=0  TranslationLengthUnit=m  TranslationStandardAxis=+Z  TranslationCartesianOffset=[0 0 0]  TranslationROffset=0  TranslationROffsetUnits=m  TranslationZOffset=0  TranslationZOffsetUnits=m  TranslationThetaOffset=0  TranslationThetaOffsetUnits=deg  RotationMethod=StandardAxis  RotationAngleUnits=deg  RotationStandardAxis=+Z  RotationAngle=180  RotationArbitraryAxis=[0 0 1]  FollAlignAxisA=+X  BaseAlignAxisA=+Y  FollAlignAxisB=+Y  BaseAlignAxisB=+Z  RotationSequenceAxes=FollowerAxes  RotationSequence=XYX  RotationSequenceAngles=[0 0 0]  RotationSequenceAnglesUnits=deg  RotationMatrix=[1 0 0; 0 1 0; 0 0 1]
  Rigid Transform1 : sm_lib/Frames and Transforms/Rigid Transform  TranslationMethod=None  TranslationStandardOffset=0  TranslationLengthUnit=m  TranslationStandardAxis=+Z  TranslationCartesianOffset=[0 0 0]  TranslationROffset=0  TranslationROffsetUnits=m  TranslationZOffset=0  TranslationZOffsetUnits=m  TranslationThetaOffset=0  TranslationThetaOffsetUnits=deg  RotationMethod=StandardAxis  RotationAngleUnits=deg  RotationStandardAxis=+Z  RotationAngle=180  RotationArbitraryAxis=[0 0 1]  FollAlignAxisA=+X  BaseAlignAxisA=+Y  FollAlignAxisB=+Y  BaseAlignAxisB=+Z  RotationSequenceAxes=FollowerAxes  RotationSequence=XYX  RotationSequenceAngles=[0 0 0]  RotationSequenceAnglesUnits=deg  RotationMatrix=[1 0 0; 0 1 0; 0 0 1]
  Rigid Transform2 : sm_lib/Frames and Transforms/Rigid Transform  TranslationMethod=None  TranslationStandardOffset=0  TranslationLengthUnit=m  TranslationStandardAxis=+Z  TranslationCartesianOffset=[0 0 0]  TranslationROffset=0  TranslationROffsetUnits=m  TranslationZOffset=0  TranslationZOffsetUnits=m  TranslationThetaOffset=0  TranslationThetaOffsetUnits=deg  RotationMethod=StandardAxis  RotationAngleUnits=deg  RotationStandardAxis=+Z  RotationAngle=180  RotationArbitraryAxis=[0 0 1]  FollAlignAxisA=+X  BaseAlignAxisA=+Y  FollAlignAxisB=+Y  BaseAlignAxisB=+Z  RotationSequenceAxes=FollowerAxes  RotationSequence=XYX  RotationSequenceAngles=[0 0 0]  RotationSequenceAnglesUnits=deg  RotationMatrix=[1 0 0; 0 1 0; 0 0 1]
  Rigid Transform3 : sm_lib/Frames and Transforms/Rigid Transform  TranslationMethod=None  TranslationStandardOffset=0  TranslationLengthUnit=m  TranslationStandardAxis=+Z  TranslationCartesianOffset=[0 0 0]  TranslationROffset=0  TranslationROffsetUnits=m  TranslationZOffset=0  TranslationZOffsetUnits=m  TranslationThetaOffset=0  TranslationThetaOffsetUnits=deg  RotationMethod=StandardAxis  RotationAngleUnits=deg  RotationStandardAxis=+Z  RotationAngle=90  RotationArbitraryAxis=[0 0 1]  FollAlignAxisA=+X  BaseAlignAxisA=+Y  FollAlignAxisB=+Y  BaseAlignAxisB=+Z  RotationSequenceAxes=FollowerAxes  RotationSequence=XYX  RotationSequenceAngles=[0 0 0]  RotationSequenceAnglesUnits=deg  RotationMatrix=[1 0 0; 0 1 0; 0 0 1]
  Simulink-PS Converter{1..4} (4 alike) : nesl_utility/Simulink-PS Converter  PhysicalDomain=network_engine_domain  SubClassName=ps_input  LeftPortType=input  RightPortType=output  PseudoPeriodic=off  Frequencies=[]  NoiseDistribution=none  NoiseParameters=[]  Unit=1  AffineConversion=off  FilteringAndDerivatives=filter  SimscapeFilterOrder=2  InputFilterTimeConstant=0.001  UdotUserProvided=0
  Solver Configuration : nesl_utility/Solver Configuration  PhysicalDomain=network_engine_domain  SubClassName=solver  LeftPortType=input  RightPortType=generic  Tones=[]  Harmonics=[]  SimulateNoise=off  Profile=off  UseLocalSampling=off  EnableSwitchedLinearOptims=on  FrequencyDomain=off  UseCCode=off  RelTol=0.001  AbsTol=1e-06  MinStep=1e-09  ToWorkspace=off  RevertToSquareIcSolve=off  NumHomotopyIterations=100  PhasorMode=off  PhasorModeNumHarmonics=1  DoDC=off  ResidualTolerance=1e-09  UseLocalSolver=off  LocalSolverChoice=NE_BACKWARD_EULER_ADVANCER  LocalSolverSampleTime=0.001  DoFixedCost=off  MaxNonlinIter=3  MaxModeIter=2  LinearAlgebra=Sparse  EquationFormulation=NE_TIME_EF  DelaysMemoryBudget=1024  AutomaticFiltering=on  FilteringTimeConstant=0.001
  Tool1_1_RIGID : Subsystem
  Tool2_1_RIGID : Subsystem
  Tool2_2_RIGID : Subsystem
  Transform Sensor2 : sm_lib/Frames and Transforms/Transform Sensor  MeasurementFrame=World  SenseAngle=off  SenseAxis=off  SenseAngle1=off  SenseAngle2=off  SenseAngle3=off  SenseQ=off  SenseR=off  SenseOmegaX=off  SenseOmegaY=off  SenseOmegaZ=off  SenseOmega1=off  SenseOmega2=off  SenseOmega3=off  SenseQDot=off  SenseRDot=off  SenseAlphaX=off  SenseAlphaY=off  SenseAlphaZ=off  SenseAlpha1=off  SenseAlpha2=off  SenseAlpha3=off  SenseQDDot=off  SenseRDDot=off  SenseX=on  SenseY=on  SenseZ=on  SenseRad=off  SenseAzim=off  SenseDist=off  SenseInc=off  SenseXDot=off  SenseYDot=off  SenseZDot=off  SenseRadDot=off  SenseAzimDot=off  SenseDistDot=off  SenseIncDot=off  SenseXDDot=off  SenseYDDot=off  SenseZDDot=off  SenseRadDDot=off  SenseAzimDDot=off  SenseDistDDot=off  SenseIncDDot=off
  Transform1 : sm_lib/Frames and Transforms/Rigid Transform  TranslationMethod=Cartesian  TranslationStandardOffset=0  TranslationLengthUnit=mm  TranslationStandardAxis=+Z  TranslationCartesianOffset=smiData.RigidTransform(14).translation  TranslationROffset=0  TranslationROffsetUnits=m  TranslationZOffset=0  TranslationZOffsetUnits=m  TranslationThetaOffset=0  TranslationThetaOffsetUnits=deg  RotationMethod=ArbitraryAxis  RotationAngleUnits=rad  RotationStandardAxis=+Z  RotationAngle=smiData.RigidTransform(14).angle  RotationArbitraryAxis=smiData.RigidTransform(14).axis  FollAlignAxisA=+X  BaseAlignAxisA=+Y  FollAlignAxisB=+Y  BaseAlignAxisB=+Z  RotationSequenceAxes=FollowerAxes  RotationSequence=XYX  RotationSequenceAngles=[0 0 0]  RotationSequenceAnglesUnits=deg  RotationMatrix=[1 0 0; 0 1 0; 0 0 1]
  Transform2 : sm_lib/Frames and Transforms/Rigid Transform  TranslationMethod=Cartesian  TranslationStandardOffset=0  TranslationLengthUnit=mm  TranslationStandardAxis=+Z  TranslationCartesianOffset=smiData.RigidTransform(21).translation  TranslationROffset=0  TranslationROffsetUnits=m  TranslationZOffset=0  TranslationZOffsetUnits=m  TranslationThetaOffset=0  TranslationThetaOffsetUnits=deg  RotationMethod=ArbitraryAxis  RotationAngleUnits=rad  RotationStandardAxis=+Z  RotationAngle=smiData.RigidTransform(21).angle  RotationArbitraryAxis=smiData.RigidTransform(21).axis  FollAlignAxisA=+X  BaseAlignAxisA=+Y  FollAlignAxisB=+Y  BaseAlignAxisB=+Z  RotationSequenceAxes=FollowerAxes  RotationSequence=XYX  RotationSequenceAngles=[0 0 0]  RotationSequenceAnglesUnits=deg  RotationMatrix=[1 0 0; 0 1 0; 0 0 1]
  Transform3 : sm_lib/Frames and Transforms/Rigid Transform  TranslationMethod=Cartesian  TranslationStandardOffset=0  TranslationLengthUnit=mm  TranslationStandardAxis=+Z  TranslationCartesianOffset=smiData.RigidTransform(22).translation  TranslationROffset=0  TranslationROffsetUnits=m  TranslationZOffset=0  TranslationZOffsetUnits=m  TranslationThetaOffset=0  TranslationThetaOffsetUnits=deg  RotationMethod=ArbitraryAxis  RotationAngleUnits=rad  RotationStandardAxis=+Z  RotationAngle=smiData.RigidTransform(22).angle  RotationArbitraryAxis=smiData.RigidTransform(22).axis  FollAlignAxisA=+X  BaseAlignAxisA=+Y  FollAlignAxisB=+Y  BaseAlignAxisB=+Z  RotationSequenceAxes=FollowerAxes  RotationSequence=XYX  RotationSequenceAngles=[0 0 0]  RotationSequenceAnglesUnits=deg  RotationMatrix=[1 0 0; 0 1 0; 0 0 1]
  Transform4 : sm_lib/Frames and Transforms/Rigid Transform  TranslationMethod=Cartesian  TranslationStandardOffset=0  TranslationLengthUnit=mm  TranslationStandardAxis=+Z  TranslationCartesianOffset=smiData.RigidTransform(23).translation  TranslationROffset=0  TranslationROffsetUnits=m  TranslationZOffset=0  TranslationZOffsetUnits=m  TranslationThetaOffset=0  TranslationThetaOffsetUnits=deg  RotationMethod=ArbitraryAxis  RotationAngleUnits=rad  RotationStandardAxis=+Z  RotationAngle=smiData.RigidTransform(23).angle  RotationArbitraryAxis=smiData.RigidTransform(23).axis  FollAlignAxisA=+X  BaseAlignAxisA=+Y  FollAlignAxisB=+Y  BaseAlignAxisB=+Z  RotationSequenceAxes=FollowerAxes  RotationSequence=XYX  RotationSequenceAngles=[0 0 0]  RotationSequenceAnglesUnits=deg  RotationMatrix=[1 0 0; 0 1 0; 0 0 1]
  World : sm_lib/Frames and Transforms/World Frame
  X : Outport  VectorParamsAs1DForOutWhenUnconnected=on
  Y : Outport  Port=2  VectorParamsAs1DForOutWhenUnconnected=on
  Z : Outport  Port=3  VectorParamsAs1DForOutWhenUnconnected=on
  q1 : Outport  Port=4  VectorParamsAs1DForOutWhenUnconnected=on
  q2 : Outport  Port=5  VectorParamsAs1DForOutWhenUnconnected=on
  q3 : Outport  Port=6  VectorParamsAs1DForOutWhenUnconnected=on
  w1 : Outport  Port=7  VectorParamsAs1DForOutWhenUnconnected=on
  w2 : Outport  Port=8  VectorParamsAs1DForOutWhenUnconnected=on
  w3 : Outport  Port=9  VectorParamsAs1DForOutWhenUnconnected=on
  T1 : Outport  Port=10  VectorParamsAs1DForOutWhenUnconnected=on
  T2 : Outport  Port=11  VectorParamsAs1DForOutWhenUnconnected=on
  T3 : Outport  Port=12  VectorParamsAs1DForOutWhenUnconnected=on
  q4 : Outport  Port=13  VectorParamsAs1DForOutWhenUnconnected=on
  wires:
  Th2/1 -> Simulink-PS Converter1/1
  Th3/1 -> Simulink-PS Converter2/1
  Th1/1 -> Simulink-PS Converter3/1
  PS-Simulink Converter/1 -> X/1
  PS-Simulink Converter1/1 -> Y/1
  PS-Simulink Converter2/1 -> Z/1
  PS-Simulink Converter3/1 -> q1/1
  PS-Simulink Converter4/1 -> q2/1
  PS-Simulink Converter5/1 -> q3/1
  PS-Simulink Converter6/1 -> w1/1
  PS-Simulink Converter7/1 -> w2/1
  PS-Simulink Converter8/1 -> w3/1
  PS-Simulink Converter9/1 -> T1/1
  PS-Simulink Converter10/1 -> T2/1
  PS-Simulink Converter11/1 -> T3/1
  PS-Simulink Converter12/1 -> q4/1
  Th4/1 -> Simulink-PS Converter4/1
  connections:
  Base_1_RIGID/LConn1 -- Transform Sensor2/LConn1 -- Transform1/RConn1
  Link3_1_RIGID/LConn1 -- Rigid Transform1/RConn1
  R5/RConn1 -- Rigid Transform3/LConn1
  Rigid Transform2/RConn1 -- Link4_1_RIGID/LConn1
  Base_1_RIGID/RConn2 -- Plane_1_RIGID/LConn1
  Rigid Transform/RConn1 -- Link2_1_RIGID/LConn1
  Transform2/LConn1 -- Transform1/LConn1 -- MechanismConfiguration/RConn1 -- Solver Configuration/RConn1 -- World/RConn1 -- Transform3/LConn1 -- Transform4/LConn1
  R2/RConn1 -- Link1_1_RIGID/RConn1
  Link2_1_RIGID/RConn1 -- R3/LConn1
  Rigid Transform1/LConn1 -- R3/RConn1
  Simulink-PS Converter1/RConn1 -- R2/LConn2
  Link1_1_RIGID/LConn1 -- R1/RConn1
  Prismatic/RConn1 -- Tool2_1_RIGID/LConn1
  Prismatic/LConn1 -- Tool1_1_RIGID/RConn2
  R4/LConn1 -- Rigid Transform2/LConn1
  Base_1_RIGID/RConn1 -- R1/LConn1
  R2/LConn1 -- Rigid Transform/LConn1
  R4/RConn1 -- Link3_1_RIGID/RConn1
  R5/LConn1 -- Link4_1_RIGID/RConn1
  Simulink-PS Converter3/RConn1 -- R1/LConn2
  Prismatic1/RConn1 -- Tool1_1_RIGID/RConn1
  Rigid Transform3/RConn1 -- Tool1_1_RIGID/LConn1
  Simulink-PS Converter2/RConn1 -- R3/LConn2
  Prismatic1/LConn1 -- Tool2_2_RIGID/LConn1
  Transform Sensor2/RConn1 -- Tool2_2_RIGID/LConn2
  PS-Simulink Converter/LConn1 -- Transform Sensor2/RConn2
  PS-Simulink Converter1/LConn1 -- Transform Sensor2/RConn3
  PS-Simulink Converter2/LConn1 -- Transform Sensor2/RConn4
  PS-Simulink Converter3/LConn1 -- R1/RConn2
  PS-Simulink Converter4/LConn1 -- R2/RConn2
  PS-Simulink Converter5/LConn1 -- R3/RConn2
  PS-Simulink Converter6/LConn1 -- R1/RConn3
  PS-Simulink Converter7/LConn1 -- R2/RConn3
  PS-Simulink Converter8/LConn1 -- R3/RConn3
  R1/RConn4 -- PS-Simulink Converter9/LConn1
  R3/RConn4 -- PS-Simulink Converter11/LConn1
  R4/RConn2 -- PS-Simulink Converter12/LConn1
  PS-Simulink Converter10/LConn1 -- R2/RConn4
  Simulink-PS Converter4/RConn1 -- R4/LConn2

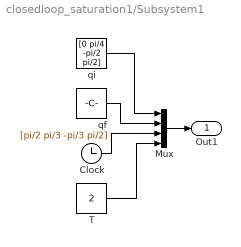
== system closedloop_saturation1/Subsystem1 ==
  Clock : Clock
  Mux : Mux
  T : Constant  Value=2
  qf : Constant  Value=[pi/2 pi/3 -pi/3 pi/2]
  qi : Constant  Value=[0 pi/4 -pi/2 pi/2]
  Out1 : Outport
  wires:
  T/1 -> Mux/4
  qi/1 -> Mux/1
  qf/1 -> Mux/2
  Clock/1 -> Mux/3
  Mux/1 -> Out1/1

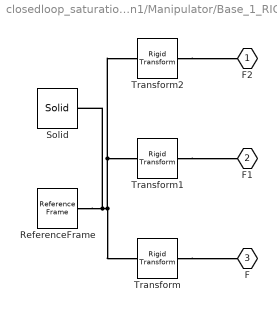
== system closedloop_saturation1/Manipulator/Base_1_RIGID ==
  ReferenceFrame : sm_lib/Frames and Transforms/Reference Frame
  Solid : sm_lib/Body Elements/Solid  InertiaType=Custom  Mass=smiData.Solid(1).mass  MassUnits=kg  CenterOfMass=smiData.Solid(1).CoM  CenterOfMassUnits=mm  MomentsOfInertia=smiData.Solid(1).MoI  MomentsOfInertiaUnits=kg*mm^2  ProductsOfInertia=smiData.Solid(1).PoI  ProductsOfInertiaUnits=kg*mm^2  DensityBased=on  Density=1000  DensityUnits=kg/m^3  DoExposeReferenceFrame=on  SerializedFrames=<Frames/>  GraphicType=FromGeometry  MarkerShape=Sphere  MarkerSize=10  GraphicVisPropType=SimpleVisualProperties  GraphicDiffuseColor=smiData.Solid(1).color  GraphicSpecularColor=[0.5 0.5 0.5 1.0]  GraphicAmbientColor=[0.15 0.15 0.15 1.0]  GraphicEmissiveColor=[0.0 0.0 0.0 1.0]  GraphicShininess=75  GraphicOpacity=smiData.Solid(1).opacity  GeometryShape=FromFile  RectangleSize=[1 1]  RectangleSizeUnits=m  BrickDimensions=[1 1 1]  BrickDimensionUnits=m  CylinderRadius=1  CylinderRadiusUnits=m  CylinderLength=1  CylinderLengthUnits=m  SphereRadius=1  SphereRadiusUnits=m  EllipsoidRadii=[1 1 1]  EllipsoidRadiiUnits=m  ExtrusionCrossSection=[1 1; -1 1; -1 -1; 1 -1]  ExtrusionCrossSectionUnits=m  ExtrusionLength=1  ExtrusionLengthUnits=m  PolygonNumSides=3  PolygonOuterRadius=1  PolygonOuterRadiusUnits=m  ExtGeomFileType=STEP  ExtGeomFileName=Base_Default_sldprt.STEP  ExtGeomFileUnits=m  RevolutionCrossSection=[1 1; 1 -1; 2 -1; 2 1]  RevolutionCrossSectionUnits=m  RevolutionExtent=Full  RevolutionAngle=180  RevolutionAngleUnits=deg
  Transform : sm_lib/Frames and Transforms/Rigid Transform  TranslationMethod=Cartesian  TranslationStandardOffset=0  TranslationLengthUnit=mm  TranslationStandardAxis=+Z  TranslationCartesianOffset=smiData.RigidTransform(1).translation  TranslationROffset=0  TranslationROffsetUnits=m  TranslationZOffset=0  TranslationZOffsetUnits=m  TranslationThetaOffset=0  TranslationThetaOffsetUnits=deg  RotationMethod=ArbitraryAxis  RotationAngleUnits=rad  RotationStandardAxis=+Z  RotationAngle=smiData.RigidTransform(1).angle  RotationArbitraryAxis=smiData.RigidTransform(1).axis  FollAlignAxisA=+X  BaseAlignAxisA=+Y  FollAlignAxisB=+Y  BaseAlignAxisB=+Z  RotationSequenceAxes=FollowerAxes  RotationSequence=XYX  RotationSequenceAngles=[0 0 0]  RotationSequenceAnglesUnits=deg  RotationMatrix=[1 0 0; 0 1 0; 0 0 1]
  Transform1 : sm_lib/Frames and Transforms/Rigid Transform  TranslationMethod=Cartesian  TranslationStandardOffset=0  TranslationLengthUnit=mm  TranslationStandardAxis=+Z  TranslationCartesianOffset=smiData.RigidTransform(7).translation  TranslationROffset=0  TranslationROffsetUnits=m  TranslationZOffset=0  TranslationZOffsetUnits=m  TranslationThetaOffset=0  TranslationThetaOffsetUnits=deg  RotationMethod=ArbitraryAxis  RotationAngleUnits=rad  RotationStandardAxis=+Z  RotationAngle=smiData.RigidTransform(7).angle  RotationArbitraryAxis=smiData.RigidTransform(7).axis  FollAlignAxisA=+X  BaseAlignAxisA=+Y  FollAlignAxisB=+Y  BaseAlignAxisB=+Z  RotationSequenceAxes=FollowerAxes  RotationSequence=XYX  RotationSequenceAngles=[0 0 0]  RotationSequenceAnglesUnits=deg  RotationMatrix=[1 0 0; 0 1 0; 0 0 1]
  Transform2 : sm_lib/Frames and Transforms/Rigid Transform  TranslationMethod=Cartesian  TranslationStandardOffset=0  TranslationLengthUnit=mm  TranslationStandardAxis=+Z  TranslationCartesianOffset=smiData.RigidTransform(13).translation  TranslationROffset=0  TranslationROffsetUnits=m  TranslationZOffset=0  TranslationZOffsetUnits=m  TranslationThetaOffset=0  TranslationThetaOffsetUnits=deg  RotationMethod=ArbitraryAxis  RotationAngleUnits=rad  RotationStandardAxis=+Z  RotationAngle=smiData.RigidTransform(13).angle  RotationArbitraryAxis=smiData.RigidTransform(13).axis  FollAlignAxisA=+X  BaseAlignAxisA=+Y  FollAlignAxisB=+Y  BaseAlignAxisB=+Z  RotationSequenceAxes=FollowerAxes  RotationSequence=XYX  RotationSequenceAngles=[0 0 0]  RotationSequenceAnglesUnits=deg  RotationMatrix=[1 0 0; 0 1 0; 0 0 1]
  F2 : PMIOPort  Side=Left
  F1 : PMIOPort  Port=2  Side=Right
  F : PMIOPort  Port=3  Side=Right
  connections:
  Solid/RConn1 -- ReferenceFrame/RConn1 -- Transform1/LConn1 -- Transform2/LConn1 -- Transform/LConn1
  Transform/RConn1 -- F/RConn1
  Transform1/RConn1 -- F1/RConn1
  Transform2/RConn1 -- F2/RConn1
